simulink model "Boomerang_Simulink_Nav_Kalman"  (R2023a)
settings: Solver=ode4  StartTime=0.0  StopTime=t  FixedStep=dt  MaxStep=maxstep  MinStep=minstep
values from neighbouring files (symbols this model uses):
  c = 5e-2    (= 0.05)    [Boomerang_4Wings.m]    (also in Boomerang_4Wings_Titan.m = 0.0488; Boomerang_4Wings_Venus52.m; Boomerang_4Wings_Venus60.m = 0.065; Boomerang_Cropped_Validation.m = 0.0381)
  CDdata = [x_CD, y_CD]    [Boomerang_4Wings.m]    (also in Boomerang_4Wings_Titan.m; Boomerang_4Wings_Venus52.m; Boomerang_4Wings_Venus60.m; Boomerang_Cropped_Validation.m)
  CLdata = [x_CL, y_CL]    [Boomerang_4Wings.m]    (also in Boomerang_4Wings_Titan.m; Boomerang_4Wings_Venus52.m; Boomerang_4Wings_Venus60.m; Boomerang_Cropped_Validation.m)
  CMdata = [x_CM, y_CM]    [Boomerang_4Wings.m]    (also in Boomerang_4Wings_Titan.m; Boomerang_4Wings_Venus52.m; Boomerang_4Wings_Venus60.m; Boomerang_Cropped_Validation.m)
  dt = 2e-4    (= 0.0002)    [Boomerang_4Wings.m]    (also in Boomerang_4Wings_Titan.m; Boomerang_4Wings_Venus52.m; Boomerang_4Wings_Venus60.m; Boomerang_Cropped_Validation.m)
  Eul0 = [0; 0; 0]    [Boomerang_4Wings.m]    (also in Boomerang_4Wings_Titan.m; Boomerang_4Wings_Venus52.m; Boomerang_4Wings_Venus60.m; Boomerang_Cropped_Validation.m)
  f = 1000    [Boomerang_4Wings.m]    (also in Boomerang_Flight_Dynamics.m; Boomerang_Flight_Dynamics_twisted_wing.m = @(x) -sqrt(abs(Rp^2 - (x-a(2)).^2)) + b(2); Plot_Results.m = @(x) -sqrt(abs(Rp^2 - (x-a(2)).^2)) + b(2); Vassberg.mat = )
  g = 9.81    [Boomerang_4Wings.m]    (also in Boomerang_4Wings_Titan.m = 1.35; Boomerang_4Wings_Venus52.m; Boomerang_4Wings_Venus60.m = 8.87; Boomerang_Cropped_Validation.m)
  h = l_blade/n    (= 0.006)    [Boomerang_Flight_Dynamics.m]    (also in Boomerang_Flight_Dynamics_twisted_wing.m; Vassberg.mat)
  invJ = inv(J)    [Boomerang_4Wings.m]    (also in Boomerang_4Wings_Titan.m; Boomerang_4Wings_Venus52.m; Boomerang_4Wings_Venus60.m; Boomerang_Cropped_Validation.m)
  invTI0 = transpose(TI0)    [AttitudePlot.m]    (also in AttitudePlot_V0.m = T; Boomerang_4Wings.m; Boomerang_4Wings_Titan.m; Boomerang_4Wings_Venus52.m)
  invTj = zeros(3,3,nw)    [Boomerang_4Wings.m]    (also in Boomerang_4Wings_Titan.m; Boomerang_4Wings_Venus52.m; Boomerang_4Wings_Venus60.m; Boomerang_Cropped_Validation.m)
  J = J + (Ji(:,:,i))    [Boomerang_4Wings.m]    (also in Boomerang_4Wings_Titan.m = diag(diag(J)); Boomerang_4Wings_Venus52.m; Boomerang_4Wings_Venus60.m; Boomerang_Cropped_Validation.m = [Ixx Ixy Ixz)
  l_integrate = linspace(0,l_blade,n)    [Boomerang_4Wings.m]    (also in Boomerang_4Wings_Titan.m; Boomerang_4Wings_Venus52.m; Boomerang_4Wings_Venus60.m; Boomerang_Cropped_Validation.m = linspace(l_blade_0,l_blade,n))
  m = m_b    (= 0.2)    [Boomerang_4Wings.m]    (also in Boomerang_4Wings_Titan.m = m_b*eye(3) + m_add; Boomerang_4Wings_Venus52.m = m_b*eye(3) + m_add; Boomerang_4Wings_Venus60.m = m_b*eye(3) + m_add; Boomerang_Cropped_Validation.m = m_b*eye(3) + m_add)
  nw = 4    [Boomerang_4Wings.m]    (also in Boomerang_4Wings_Titan.m; Boomerang_4Wings_Venus52.m; Boomerang_4Wings_Venus60.m; Boomerang_Cropped_Validation.m = 3)
  omega0 = [0; 0; 10*pi*2]    [Boomerang_4Wings.m]    (also in Boomerang_4Wings_Titan.m = [0; 0; r*pi*2]; Boomerang_4Wings_Venus52.m; Boomerang_4Wings_Venus60.m; Boomerang_Cropped_Validation.m = [0; 0; r])
  PHI0 = deg2rad(PHI0)    [AttitudePlot.m]    (also in AttitudePlot_V0.m; Boomerang_4Wings.m; Boomerang_4Wings_Titan.m; Boomerang_4Wings_Venus52.m)
  PSI0 = deg2rad(PSI0)    [AttitudePlot.m]    (also in AttitudePlot_V0.m; Boomerang_4Wings.m; Boomerang_4Wings_Titan.m; Boomerang_4Wings_Venus52.m)
  R_pos0 = [0; 0; 1.5]    [Boomerang_4Wings.m]    (also in Boomerang_4Wings_Titan.m; Boomerang_4Wings_Venus52.m; Boomerang_4Wings_Venus60.m; Boomerang_Cropped_Validation.m = [0; 0; 1.8])
  rho = 1.22    [Boomerang_4Wings.m]    (also in Boomerang_4Wings_Titan.m = 5.368; Boomerang_4Wings_Venus52.m = 1.3288004; Boomerang_4Wings_Venus60.m = 0.49007955; Boomerang_Cropped_Validation.m)
  S = pi*R^2    (= 0.196349540849)    [Boomerang_4Wings.m]    (also in Boomerang_4Wings_Titan.m = 0.228; Boomerang_4Wings_Venus52.m; Boomerang_4Wings_Venus60.m = 0.282743338823; Boomerang_Cropped_Validation.m = 0.0651440652648)
  THETA0 = deg2rad(THETA0)    [AttitudePlot.m]    (also in AttitudePlot_V0.m; Boomerang_4Wings.m; Boomerang_4Wings_Titan.m; Boomerang_4Wings_Venus52.m)
  thetaj = 0    [Boomerang_4Wings.m]    (also in Boomerang_4Wings_Titan.m; Boomerang_4Wings_Venus52.m; Boomerang_4Wings_Venus60.m; Boomerang_Cropped_Validation.m = deg2rad(thetaj))
  TI0 = RI01*RI02*RI03    [AttitudePlot.m]    (also in Boomerang_4Wings.m; Boomerang_4Wings_Titan.m; Boomerang_4Wings_Venus52.m; Boomerang_4Wings_Venus60.m)
  Tj = zeros(3,3, nw)    [Boomerang_4Wings.m]    (also in Boomerang_4Wings_Titan.m; Boomerang_4Wings_Venus52.m; Boomerang_4Wings_Venus60.m; Boomerang_Cropped_Validation.m)
  u0 = TI0*U0    [Boomerang_4Wings.m]    (also in Boomerang_4Wings_Titan.m; Boomerang_4Wings_Venus52.m; Boomerang_4Wings_Venus60.m; Boomerang_Cropped_Validation.m)
  v_wind = [0; 0; 0]    [Boomerang_4Wings.m]    (also in Boomerang_4Wings_Titan.m; Boomerang_4Wings_Venus52.m; Boomerang_4Wings_Venus60.m; Boomerang_Cropped_Validation.m)
  x_ac = zeros(3,nw)    [Boomerang_4Wings.m]    (also in Boomerang_4Wings_Titan.m = 0; Boomerang_4Wings_Venus52.m; Boomerang_4Wings_Venus60.m; Boomerang_Cropped_Validation.m)
undefined symbols (not defined in the file or in its folder): delta_theta, t_action
libraries: simulink_extras x3, aerolibnav x2, sharedTrackingLibrary x2
settings Model: Creator=dsantis  LastModifiedBy=dsantis

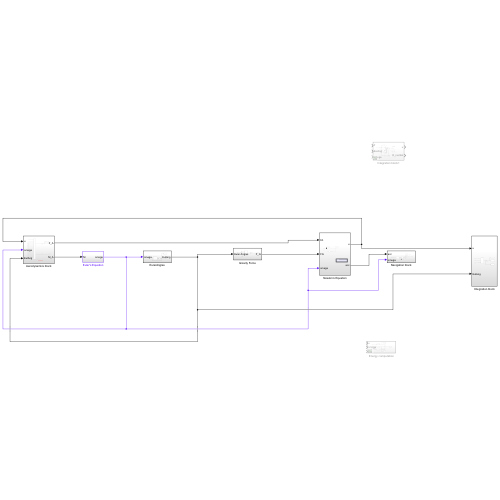
[thumbnail: Simulink's stored preview of the top-level diagram]
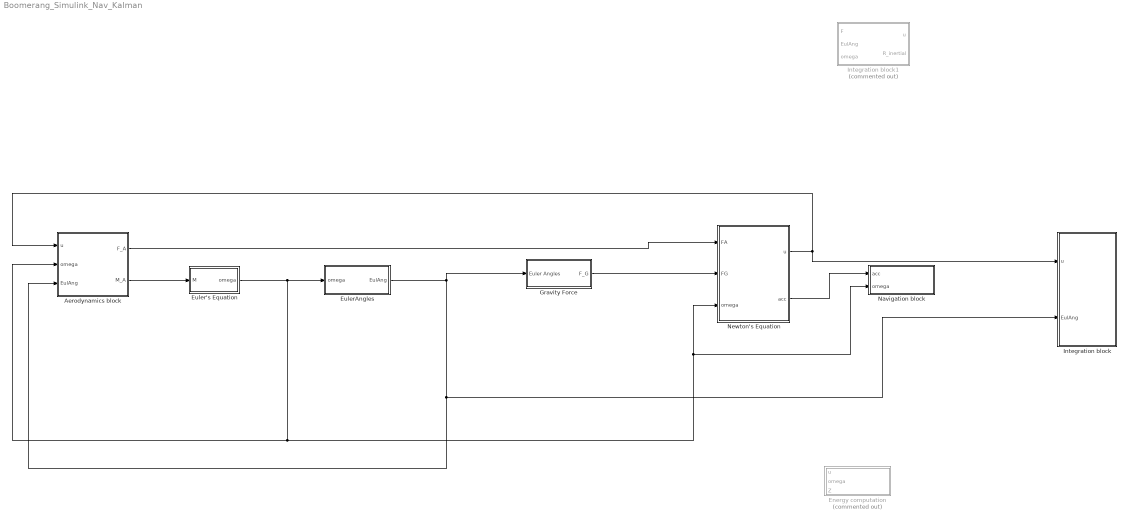
== system Boomerang_Simulink_Nav_Kalman ==
  Aerodynamics block : Subsystem
  Energy computation : Subsystem  Commented=on
  Euler's Equation : Subsystem
  EulerAngles : Subsystem
  Gravity Force : Subsystem
  Integration block : Subsystem
  Integration block1 : Subsystem  Commented=on
  Navigation block : Subsystem
  Newton's Equation : Subsystem
  wires:
  Euler's Equation/1(omega) -> EulerAngles/1(omega), Aerodynamics block/2(omega), Newton's Equation/3(omega), Navigation block/2(omega)
  Newton's Equation/1(u) -> Aerodynamics block/1(u), Integration block/1(u)
  Gravity Force/1(F_G) -> Newton's Equation/2(FG)
  Aerodynamics block/2(M_A) -> Euler's Equation/1(M)
  EulerAngles/1(EulAng) -> Gravity Force/1(Euler Angles), Aerodynamics block/3(EulAng), Integration block/2(EulAng)
  Aerodynamics block/1(F_A) -> Newton's Equation/1(FA)
  Newton's Equation/2(acc) -> Navigation block/1(acc)

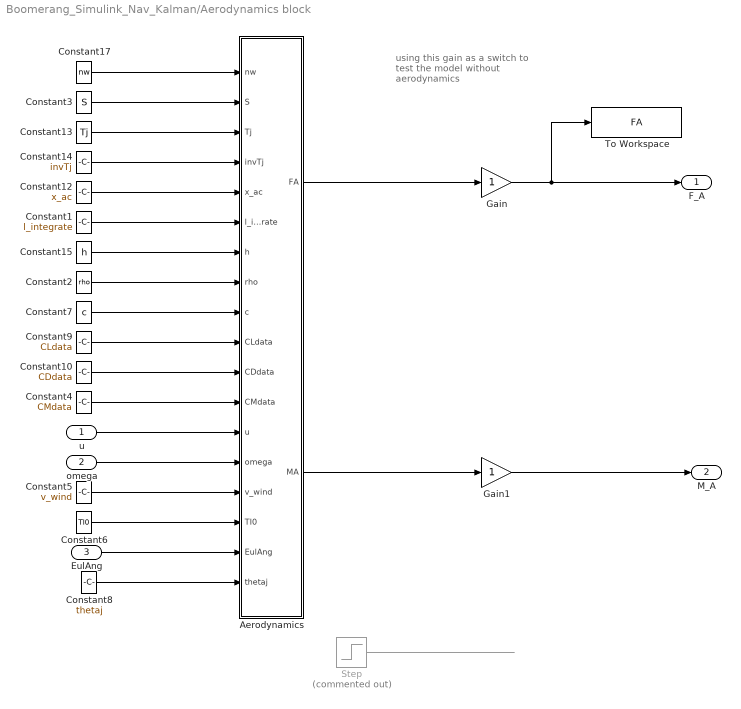
== system Boomerang_Simulink_Nav_Kalman/Aerodynamics block ==
  note: using this gain as a switch
      | to test the model without aerodynamics
  u : Inport
  omega : Inport  Port=2
  EulAng : Inport  Port=3
  Aerodynamics : MATLAB Function  TreatAsAtomicUnit=on
  Constant1 : Constant  Value=l_integrate
  Constant10 : Constant  Value=CDdata
  Constant12 : Constant  Value=x_ac
  Constant13 : Constant  Value=Tj
  Constant14 : Constant  Value=invTj
  Constant15 : Constant  Value=h
  Constant17 : Constant  Value=nw
  Constant2 : Constant  Value=rho
  Constant3 : Constant  Value=S
  Constant4 : Constant  Value=CMdata
  Constant5 : Constant  Value=v_wind
  Constant6 : Constant  Value=TI0
  Constant7 : Constant  Value=c
  Constant8 : Constant  Value=thetaj
  Constant9 : Constant  Value=CLdata
  Gain : Gain
  Gain1 : Gain
  Step : Step  Commented=on  Time=t_action  After=delta_theta  SampleTime=0  VectorParams1D=off
  To Workspace : ToWorkspace  VariableName=FA  SaveFormat=Timeseries  SampleTime=-1
  F_A : Outport
  M_A : Outport  Port=2
  wires:
  u/1 -> Aerodynamics/13(u)
  Constant2/1 -> Aerodynamics/8(rho)
  Constant9/1 -> Aerodynamics/10(CLdata)
  Constant10/1 -> Aerodynamics/11(CDdata)
  Constant1/1 -> Aerodynamics/6(l_integrate)
  Constant7/1 -> Aerodynamics/9(c)
  omega/1 -> Aerodynamics/14(omega)
  Constant12/1 -> Aerodynamics/5(x_ac)
  Constant14/1 -> Aerodynamics/4(invTj)
  Constant13/1 -> Aerodynamics/3(Tj)
  Constant15/1 -> Aerodynamics/7(h)
  Aerodynamics/1(FA) -> Gain/1
  Constant17/1 -> Aerodynamics/1(nw)
  Constant3/1 -> Aerodynamics/2(S)
  Gain/1 -> To Workspace/1, F_A/1
  Constant4/1 -> Aerodynamics/12(CMdata)
  Gain1/1 -> M_A/1
  Step/1 -> ?
  Aerodynamics/2(MA) -> Gain1/1
  Constant5/1 -> Aerodynamics/15(v_wind)
  Constant6/1 -> Aerodynamics/16(TI0)
  EulAng/1 -> Aerodynamics/17(EulAng)
  Constant8/1 -> Aerodynamics/18(thetaj)

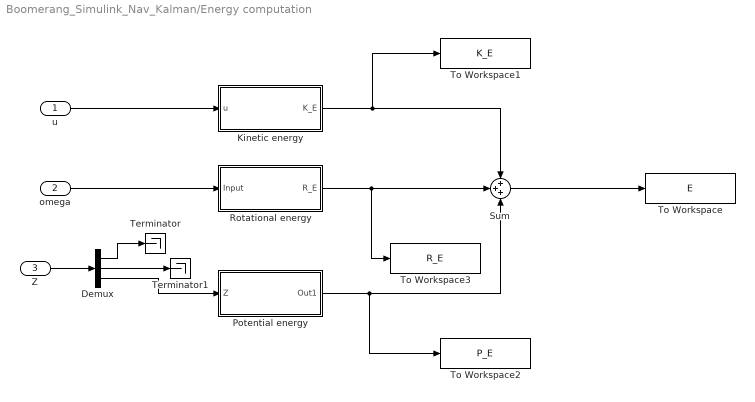
== system Boomerang_Simulink_Nav_Kalman/Energy computation ==
  u : Inport
  omega : Inport  Port=2
  Z : Inport  Port=3
  Demux : Demux  Outputs=3
  Kinetic energy : Subsystem
  Potential energy : Subsystem
  Rotational energy : Subsystem
  Sum : Sum  Inputs=+++
  Terminator : Terminator
  Terminator1 : Terminator
  To Workspace : ToWorkspace  VariableName=E  SaveFormat=Timeseries  SampleTime=-1
  To Workspace1 : ToWorkspace  VariableName=K_E  SaveFormat=Timeseries  SampleTime=-1
  To Workspace2 : ToWorkspace  VariableName=P_E  SaveFormat=Timeseries  SampleTime=-1
  To Workspace3 : ToWorkspace  VariableName=R_E  SaveFormat=Timeseries  SampleTime=-1
  wires:
  u/1 -> Kinetic energy/1(u)
  omega/1 -> Rotational energy/1(Input)
  Z/1 -> Demux/1
  Demux/3 -> Potential energy/1(Z)
  Demux/1 -> Terminator/1
  Demux/2 -> Terminator1/1
  Kinetic energy/1(K_E) -> To Workspace1/1, Sum/1
  Rotational energy/1(R_E) -> To Workspace3/1, Sum/2
  Potential energy/1(Out1) -> To Workspace2/1, Sum/3
  Sum/1 -> To Workspace/1

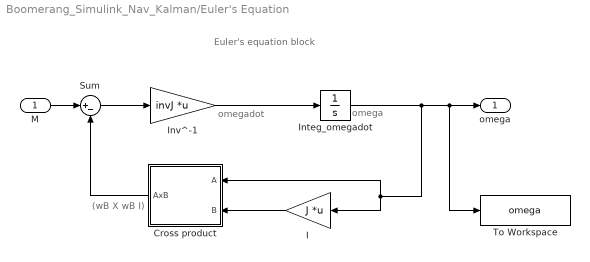
== system Boomerang_Simulink_Nav_Kalman/Euler's Equation ==
  note: Euler's equation block
  note: (wB X wB I)
  note: omega
  note: omegadot
  M : Inport
  Cross product : Subsystem
  I : Gain  Gain=J  Multiplication=Matrix(K*u)
  Integ_omegadot : Integrator  InitialCondition=omega0
  Inv^-1 : Gain  Gain=invJ  Multiplication=Matrix(K*u) (u vector)
  Sum : Sum  Inputs=|+-
  To Workspace : ToWorkspace  VariableName=omega  SampleTime=-1
  omega : Outport  VectorParamsAs1DForOutWhenUnconnected=off
  wires:
  Integ_omegadot/1 -> To Workspace/1, omega/1, I/1, Cross product/1(A)
  I/1 -> Cross product/2(B)
  M/1 -> Sum/1
  Sum/1 -> Inv^-1/1
  Inv^-1/1 -> Integ_omegadot/1
  Cross product/1(AxB) -> Sum/2

== system Boomerang_Simulink_Nav_Kalman/EulerAngles ==
  omega : Inport
  Integrator : Integrator  InitialCondition=Eul0
  MATLAB Function : MATLAB Function  TreatAsAtomicUnit=on
  To Workspace : ToWorkspace  VariableName=EulAng  SampleTime=-1
  EulAng : Outport
  wires:
  omega/1 -> MATLAB Function/1(omega)
  MATLAB Function/1(EulRate) -> Integrator/1
  Integrator/1 -> MATLAB Function/2(EulAng), EulAng/1, To Workspace/1

== system Boomerang_Simulink_Nav_Kalman/Gravity Force ==
  Euler Angles : Inport
  Constant : Constant  Value=TI0
  Demux : Demux  Outputs=3
  Gain : Gain  Gain=-m*g
  MATLAB Function : MATLAB Function  TreatAsAtomicUnit=on
  F_G : Outport
  wires:
  Gain/1 -> F_G/1
  Demux/3 -> MATLAB Function/3(psi)
  Demux/2 -> MATLAB Function/2(theta)
  Demux/1 -> MATLAB Function/1(phi)
  MATLAB Function/1(CG) -> Gain/1
  Euler Angles/1 -> Demux/1
  Constant/1 -> MATLAB Function/4(TI0)

== system Boomerang_Simulink_Nav_Kalman/Integration block ==
  u : Inport
  EulAng : Inport  Port=2
  Body2Inertial : MATLAB Function  TreatAsAtomicUnit=on
  Constant : Constant  Value=invTI0
  Integrator1 : Integrator  InitialCondition=R_pos0
  Stop if Z < 0 : Subsystem
  To Workspace : ToWorkspace  VariableName=U  SampleTime=-1
  To Workspace1 : ToWorkspace  VariableName=R_inertial  SampleTime=-1
  wires:
  Integrator1/1 -> Stop if Z < 0/1(R_inertial), To Workspace1/1
  Body2Inertial/1(U) -> To Workspace/1, Integrator1/1
  u/1 -> Body2Inertial/1(u)
  Constant/1 -> Body2Inertial/3(invTI0)
  EulAng/1 -> Body2Inertial/2(EulAng)

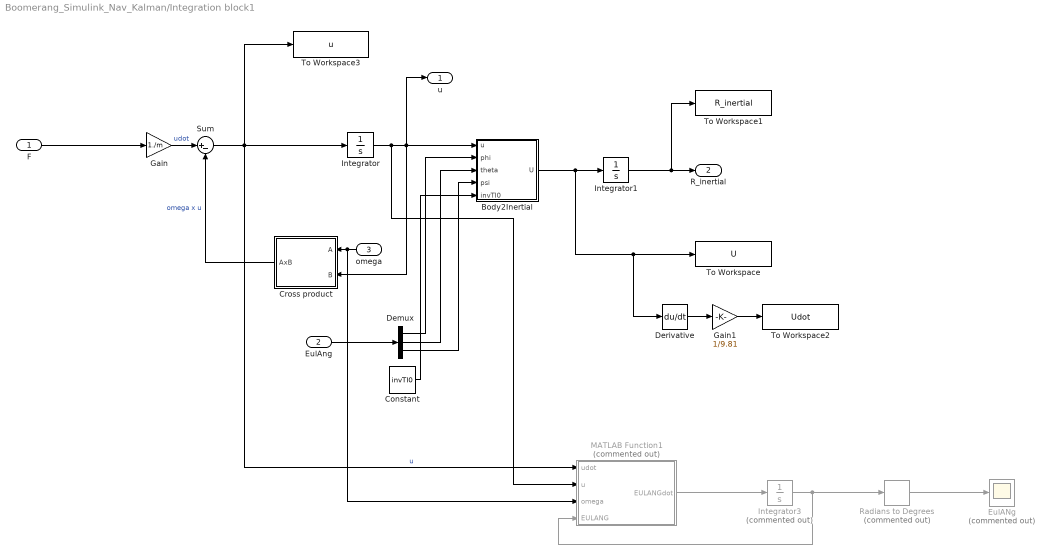
== system Boomerang_Simulink_Nav_Kalman/Integration block1 ==
  F : Inport
  EulAng : Inport  Port=2
  omega : Inport  Port=3
  Body2Inertial : MATLAB Function  TreatAsAtomicUnit=on
  Constant : Constant  Value=invTI0
  Cross product : Subsystem
  Demux : Demux  Outputs=3
  Derivative : Derivative
  EulANg : Scope  Commented=on
  Gain : Gain  Gain=1./m
  Gain1 : Gain  Gain=1/9.81
  Integrator : Integrator  InitialCondition=u0
  Integrator1 : Integrator  InitialCondition=R_pos0
  Integrator3 : Integrator  Commented=on  InitialCondition=[PHI0; THETA0; PSI0]
  MATLAB Function1 : MATLAB Function  Commented=on  TreatAsAtomicUnit=on
  Radians to Degrees : simulink_extras/Transformations/Radians to Degrees  Commented=on
  Sum : Sum  Inputs=|+-
  To Workspace : ToWorkspace  VariableName=U  SampleTime=-1
  To Workspace1 : ToWorkspace  VariableName=R_inertial  SampleTime=-1
  To Workspace2 : ToWorkspace  VariableName=Udot  SaveFormat=Timeseries  SampleTime=-1
  To Workspace3 : ToWorkspace  VariableName=u  SampleTime=-1
  u : Outport
  R_inertial : Outport  Port=2
  wires:
  Cross product/1(AxB) -> Sum/2  "omega x u"
  Integrator/1 -> Cross product/2(B), Body2Inertial/1(u), u/1, MATLAB Function1/2(u)
  Integrator1/1 -> To Workspace1/1, R_inertial/1
  Gain/1 -> Sum/1  "udot"
  EulAng/1 -> Demux/1
  Demux/1 -> Body2Inertial/2(phi)
  Demux/2 -> Body2Inertial/3(theta)
  Demux/3 -> Body2Inertial/4(psi)
  Constant/1 -> Body2Inertial/5(invTI0)
  F/1 -> Gain/1
  Body2Inertial/1(U) -> Derivative/1, To Workspace/1, Integrator1/1
  Sum/1 -> To Workspace3/1, MATLAB Function1/1(udot), Integrator/1  "u"
  MATLAB Function1/1(EULANGdot) -> Integrator3/1
  Integrator3/1 -> Radians to Degrees/1, MATLAB Function1/4(EULANG)
  Radians to Degrees/1 -> EulANg/1
  Derivative/1 -> Gain1/1
  Gain1/1 -> To Workspace2/1
  omega/1 -> MATLAB Function1/3(omega), Cross product/1(A)

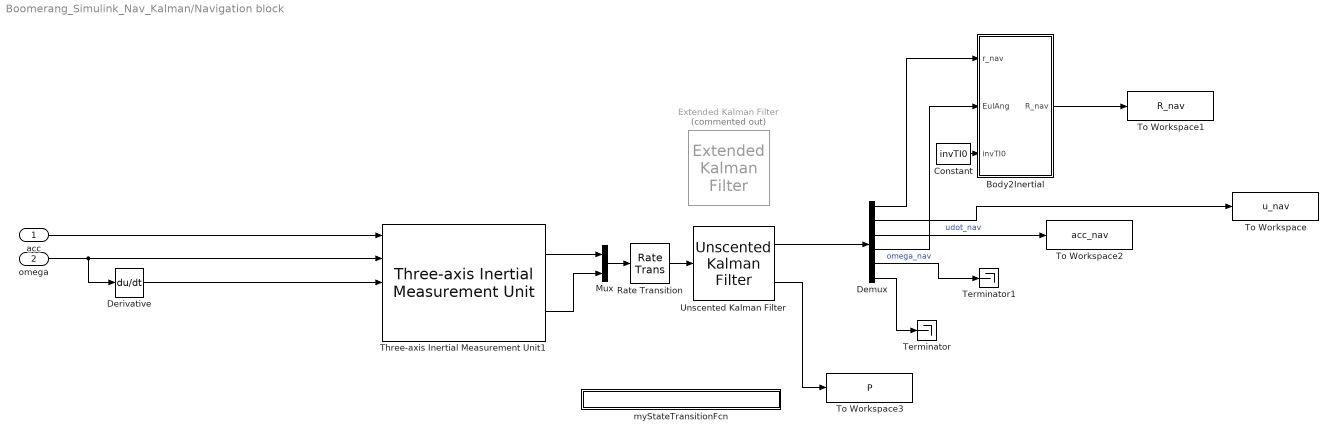
== system Boomerang_Simulink_Nav_Kalman/Navigation block ==
  acc : Inport
  omega : Inport  Port=2
  Body2Inertial : MATLAB Function  TreatAsAtomicUnit=on
  Constant : Constant  Value=invTI0
  Demux : Demux  Outputs=6
  Derivative : Derivative
  Extended Kalman Filter : sharedTrackingLibrary/Extended Kalman Filter  Commented=on  StateTransitionFcn=myStateTransitionFcn  HasStateTransitionJacobianFcn=off  HasAdditiveProcessNoise=Additive  ProcessNoise=diag(ones(18,1))  HasTimeVaryingProcessNoise=off  HasStateTransitionFcnExtraArgument=0  InitialState=[TI0*R_pos0; u0; 0; 0; 0; Eul0; omega0; 0; 0; 0]  InitialStateCovariance=diag(ones(18,1))  MeasurementFcn1=myMeasurementFcn  HasMeasurementJacobianFcn1=off  HasMeasurementEnablePort1=off  HasAdditiveMeasurementNoise1=Additive  MeasurementNoise1=[1 1 1 1 1 1]  HasTimeVaryingMeasurementNoise1=off  HasMeasurementFcnExtraArgument1=0  HasMeasurementWrapping1=off  MeasurementFcn2=myMeasurementFcn  HasMeasurementJacobianFcn2=off  HasMeasurementEnablePort2=off  HasAdditiveMeasurementNoise2=Additive  MeasurementNoise2=1  HasTimeVaryingMeasurementNoise2=off  HasMeasurementFcnExtraArgument2=0  HasMeasurementWrapping2=off  MeasurementFcn3=myMeasurementFcn  HasMeasurementJacobianFcn3=off  HasMeasurementEnablePort3=off  HasAdditiveMeasurementNoise3=Additive  MeasurementNoise3=1  HasTimeVaryingMeasurementNoise3=off  HasMeasurementFcnExtraArgument3=0  HasMeasurementWrapping3=off  MeasurementFcn4=myMeasurementFcn  HasMeasurementJacobianFcn4=off  HasMeasurementEnablePort4=off  HasAdditiveMeasurementNoise4=Additive  MeasurementNoise4=1  HasTimeVaryingMeasurementNoise4=off  HasMeasurementFcnExtraArgument4=0  HasMeasurementWrapping4=off  MeasurementFcn5=myMeasurementFcn  HasMeasurementJacobianFcn5=off  HasMeasurementEnablePort5=off  HasAdditiveMeasurementNoise5=Additive  MeasurementNoise5=1  HasTimeVaryingMeasurementNoise5=off  HasMeasurementFcnExtraArgument5=0  HasMeasurementWrapping5=off  EnableMultirate=on  StateTransitionFcnSampleTime=1/f  MeasurementFcn1SampleTime=1/f  MeasurementFcn2SampleTime=1  MeasurementFcn3SampleTime=1  MeasurementFcn4SampleTime=1  MeasurementFcn5SampleTime=1  UseCurrentEstimator=on  OutputStateCovariance=off  DataType=double  SampleTime=1  NumberOfMeasurements=1
  Mux : Mux  Inputs=2
  Rate Transition : RateTransition
  Terminator : Terminator
  Terminator1 : Terminator
  Three-axis Inertial Measurement Unit1 : aerolibnav/Three-axis Inertial Measurement Unit  units=Metric (MKS)  imu=[0 0 0]  i_Ts=0  dtype_a=off  w_a=190  z_a=0.707  a_sf_cc=acc.sf  a_bias=acc.bias  a_sat=acc.lim  dtype_g=off  w_g=190  z_g=0.707  g_sf_cc=gyro.sf  g_bias=gyro.bias  g_sens=gyro.gbias  g_sat=gyro.lim  i_rand=on  i_seeds=[23093 23094 23095 23096 23097 23098]  i_pow=noise
  To Workspace : ToWorkspace  VariableName=u_nav  SampleTime=-1
  To Workspace1 : ToWorkspace  VariableName=R_nav  SampleTime=-1
  To Workspace2 : ToWorkspace  VariableName=acc_nav  SampleTime=-1
  To Workspace3 : ToWorkspace  VariableName=P  SampleTime=-1
  Unscented Kalman Filter : sharedTrackingLibrary/Unscented Kalman Filter  StateTransitionFcn=myStateTransitionFcn  HasAdditiveProcessNoise=Additive  ProcessNoise=diag(ones(18,1))  HasTimeVaryingProcessNoise=off  HasStateTransitionFcnExtraArgument=0  InitialState=[TI0*R_pos0; u0; 0; 0; 0; Eul0; omega0; 0; 0; 0]  InitialStateCovariance=diag(ones(18,1))  Alpha=1e-3  Beta=2  Kappa=0  MeasurementFcn1=myMeasurementFcn  HasMeasurementEnablePort1=off  HasAdditiveMeasurementNoise1=Additive  MeasurementNoise1=[0.0001 0.0001 0.0001 0.0001 0.0001 0.0001]  HasTimeVaryingMeasurementNoise1=off  HasMeasurementFcnExtraArgument1=0  HasMeasurementWrapping1=off  MeasurementFcn2=myMeasurementFcn  HasMeasurementEnablePort2=off  HasAdditiveMeasurementNoise2=Additive  MeasurementNoise2=1  HasTimeVaryingMeasurementNoise2=off  HasMeasurementFcnExtraArgument2=0  HasMeasurementWrapping2=off  MeasurementFcn3=myMeasurementFcn  HasMeasurementEnablePort3=off  HasAdditiveMeasurementNoise3=Additive  MeasurementNoise3=1  HasTimeVaryingMeasurementNoise3=off  HasMeasurementFcnExtraArgument3=0  HasMeasurementWrapping3=off  MeasurementFcn4=myMeasurementFcn  HasMeasurementEnablePort4=off  HasAdditiveMeasurementNoise4=Additive  MeasurementNoise4=1  HasTimeVaryingMeasurementNoise4=off  HasMeasurementFcnExtraArgument4=0  HasMeasurementWrapping4=off  MeasurementFcn5=myMeasurementFcn  HasMeasurementEnablePort5=off  HasAdditiveMeasurementNoise5=Additive  MeasurementNoise5=1  HasTimeVaryingMeasurementNoise5=off  HasMeasurementFcnExtraArgument5=0  HasMeasurementWrapping5=off  EnableMultirate=on  StateTransitionFcnSampleTime=1/f  MeasurementFcn1SampleTime=1/f  MeasurementFcn2SampleTime=1  MeasurementFcn3SampleTime=1  MeasurementFcn4SampleTime=1  MeasurementFcn5SampleTime=1  UseCurrentEstimator=on  OutputStateCovariance=on  DataType=double  SampleTime=1  NumberOfMeasurements=1
      settings: LibrarySourceBlock=cstblocks/State Estimation/Unscented Kalman Filter
  myStateTransitionFcn : Subsystem  TreatAsAtomicUnit=on
  wires:
  Derivative/1 -> Three-axis Inertial Measurement Unit1/3
  acc/1 -> Three-axis Inertial Measurement Unit1/1
  Demux/3 -> To Workspace2/1  "udot_nav"
  omega/1 -> Three-axis Inertial Measurement Unit1/2, Derivative/1
  Demux/6 -> Terminator/1
  Demux/4 -> Body2Inertial/2(EulAng)
  Demux/1 -> Body2Inertial/1(r_nav)
  Demux/2 -> To Workspace/1
  Three-axis Inertial Measurement Unit1/1 -> Mux/1
  Three-axis Inertial Measurement Unit1/2 -> Mux/2
  Mux/1 -> Rate Transition/1
  Constant/1 -> Body2Inertial/3(invTI0)
  Body2Inertial/1(R_nav) -> To Workspace1/1
  Demux/5 -> Terminator1/1  "omega_nav"
  Rate Transition/1 -> Unscented Kalman Filter/1
  Unscented Kalman Filter/2 -> To Workspace3/1
  Unscented Kalman Filter/1 -> Demux/1

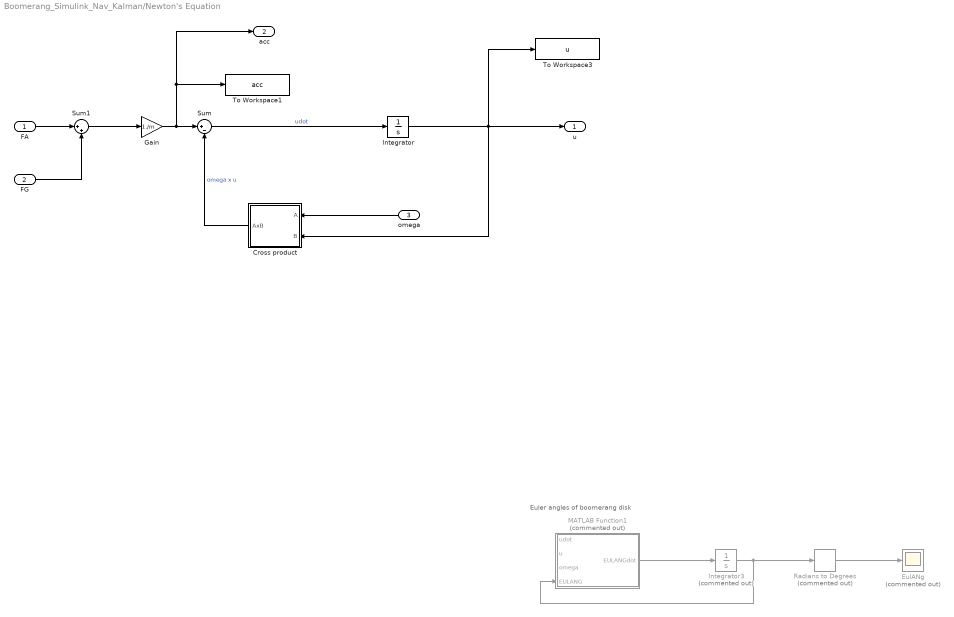
== system Boomerang_Simulink_Nav_Kalman/Newton's Equation ==
  note: Euler angles of boomerang disk
  FA : Inport
  FG : Inport  Port=2
  omega : Inport  Port=3
  Cross product : Subsystem
  EulANg : Scope  Commented=on
  Gain : Gain  Gain=1./m
  Integrator : Integrator  InitialCondition=u0
  Integrator3 : Integrator  Commented=on  InitialCondition=[PHI0; THETA0; PSI0]
  MATLAB Function1 : MATLAB Function  Commented=on  TreatAsAtomicUnit=on
  Radians to Degrees : simulink_extras/Transformations/Radians to Degrees  Commented=on
  Sum : Sum  Inputs=|+-
  Sum1 : Sum  Inputs=|++
  To Workspace1 : ToWorkspace  VariableName=acc  SampleTime=-1
  To Workspace3 : ToWorkspace  VariableName=u  SampleTime=-1
  u : Outport
  acc : Outport  Port=2
  wires:
  Cross product/1(AxB) -> Sum/2  "omega x u"
  Gain/1 -> acc/1, To Workspace1/1, Sum/1
  FA/1 -> Sum1/1
  Sum/1 -> Integrator/1  "udot"
  MATLAB Function1/1(EULANGdot) -> Integrator3/1
  Integrator3/1 -> Radians to Degrees/1, MATLAB Function1/4(EULANG)
  Radians to Degrees/1 -> EulANg/1
  omega/1 -> Cross product/1(A)
  FG/1 -> Sum1/2
  Sum1/1 -> Gain/1
  Integrator/1 -> Cross product/2(B), To Workspace3/1, u/1

== system Boomerang_Simulink_Nav_Kalman/Energy computation/Kinetic energy ==
  u : Inport
  Gain : Gain  Gain=0.5*m
  Norm : MATLAB Function  TreatAsAtomicUnit=on
  K_E : Outport
  wires:
  u/1 -> Norm/1(u)
  Norm/1(y) -> Gain/1
  Gain/1 -> K_E/1

== system Boomerang_Simulink_Nav_Kalman/Energy computation/Potential energy ==
  Z : Inport
  Gain : Gain  Gain=m*g
  Out1 : Outport
  wires:
  Z/1 -> Gain/1
  Gain/1 -> Out1/1

== system Boomerang_Simulink_Nav_Kalman/Energy computation/Rotational energy ==
  Input : Inport
  Dot Product : DotProduct  OutDataTypeStr=Inherit: Inherit via internal rule
  Gain : Gain  Gain=0.5*J  Multiplication=Matrix(u*K)
  R_E : Outport
  wires:
  Input/1 -> Dot Product/2, Gain/1
  Gain/1 -> Dot Product/1
  Dot Product/1 -> R_E/1

== system Boomerang_Simulink_Nav_Kalman/Euler's Equation/Cross product ==
  A : Inport
  B : Inport  Port=2
  MATLAB Fcn : MATLABFcn  MATLABFcn=cross(u(1:3),u(4:6))
  Mux : Mux  Inputs=2
  AxB : Outport  VectorParamsAs1DForOutWhenUnconnected=off
  wires:
  A/1 -> Mux/1
  B/1 -> Mux/2
  Mux/1 -> MATLAB Fcn/1
  MATLAB Fcn/1 -> AxB/1

== system Boomerang_Simulink_Nav_Kalman/Integration block/Stop if Z < 0 ==
  R_inertial : Inport
  Constant : Constant  Value=0
  Demux1 : Demux  Outputs=3
  Relational Operator : RelationalOperator  Operator=<=  OutDataTypeStr=boolean  RndMeth=Simplest  InputSameDT=off
  Stop Simulation : Stop
  Terminator1 : Terminator
  Terminator2 : Terminator
  Three-axis Accelerometer : aerolibnav/Three-axis Accelerometer  units=Metric (MKS)  acc=[0 0 0]  gtype=on  dtype_a=on  w_a=190  z_a=0.707  a_sf_cc=[1 0 0; 0 1 0; 0 0 1]  a_bias=[0 0 0]  a_Ts=0  a_rand=on  a_seeds=[23093 23094 23095]  a_pow=[0.001 0.001 0.001]  a_sat="[-inf  -inf  -inf  inf inf inf]"
  wires:
  R_inertial/1 -> Demux1/1
  Demux1/1 -> Terminator1/1
  Demux1/3 -> Relational Operator/1
  Demux1/2 -> Terminator2/1
  Constant/1 -> Relational Operator/2
  Relational Operator/1 -> Stop Simulation/1

== system Boomerang_Simulink_Nav_Kalman/Integration block1/Cross product ==
  A : Inport
  B : Inport  Port=2
  MATLAB Fcn : MATLABFcn  MATLABFcn=cross(u(1:3),u(4:6))
  Mux : Mux  Inputs=2
  AxB : Outport  VectorParamsAs1DForOutWhenUnconnected=off
  wires:
  A/1 -> Mux/1
  B/1 -> Mux/2
  Mux/1 -> MATLAB Fcn/1
  MATLAB Fcn/1 -> AxB/1

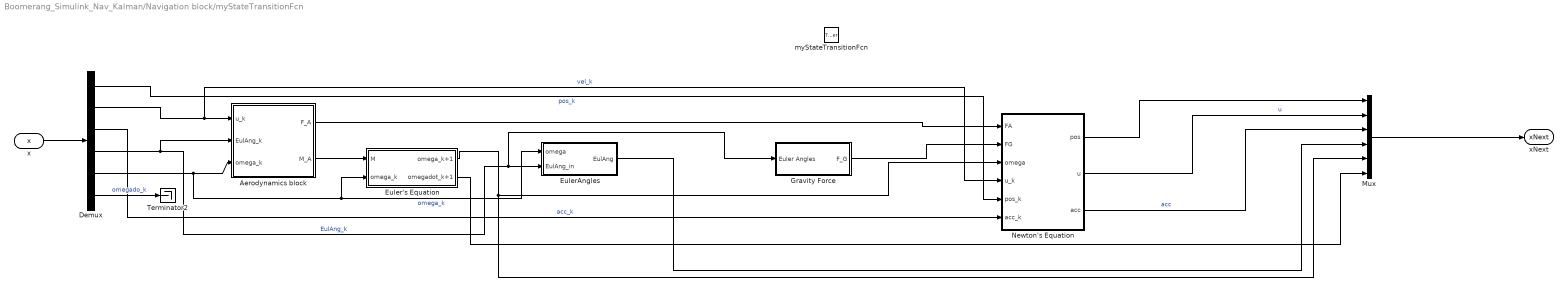
== system Boomerang_Simulink_Nav_Kalman/Navigation block/myStateTransitionFcn ==
  myStateTransitionFcn : TriggerPort  TriggerType=function-call  IsSimulinkFunction=on  FunctionName=myStateTransitionFcn  FunctionVisibility=scoped  VariantControl=(inherit)
  Aerodynamics block : Subsystem
  Demux : Demux  Outputs=6
  Euler's Equation : Subsystem
  EulerAngles : Subsystem
  Gravity Force : Subsystem
  Mux : Mux  Inputs=6
  Newton's Equation : Subsystem
  Terminator2 : Terminator
  x : ArgIn  DisableCoverage=on  PortDimensions=18  ArgumentName=x
  xNext : ArgOut  DisableCoverage=on  PortDimensions=18  ArgumentName=xNext
  wires:
  x/1 -> Demux/1
  Gravity Force/1(F_G) -> Newton's Equation/2(FG)
  EulerAngles/1(EulAng) -> Mux/4
  Aerodynamics block/1(F_A) -> Newton's Equation/1(FA)
  Aerodynamics block/2(M_A) -> Euler's Equation/1(M)
  Euler's Equation/1(omega_k+1) -> Newton's Equation/3(omega), Mux/5
  Mux/1 -> xNext/1
  Demux/1 -> Newton's Equation/5(pos_k)  "pos_k"
  Demux/2 -> Newton's Equation/4(u_k), Aerodynamics block/1(u_k)  "vel_k"
  Demux/4 -> Gravity Force/1(Euler Angles), EulerAngles/2(EulAng_in), Aerodynamics block/2(EulAng_k)  "EulAng_k"
  Demux/5 -> EulerAngles/1(omega), Euler's Equation/2(omega_k), Aerodynamics block/3(omega_k)  "omega_k"
  Demux/3 -> Newton's Equation/6(acc_k)  "acc_k"
  Demux/6 -> Terminator2/1  "omegado_k"
  Euler's Equation/2(omegadot_k+1) -> Mux/6
  Newton's Equation/2(u) -> Mux/2  "u"
  Newton's Equation/3(acc) -> Mux/3  "acc"
  Newton's Equation/1(pos) -> Mux/1

== system Boomerang_Simulink_Nav_Kalman/Newton's Equation/Cross product ==
  A : Inport
  B : Inport  Port=2
  MATLAB Fcn : MATLABFcn  MATLABFcn=cross(u(1:3),u(4:6))
  Mux : Mux  Inputs=2
  AxB : Outport  VectorParamsAs1DForOutWhenUnconnected=off
  wires:
  A/1 -> Mux/1
  B/1 -> Mux/2
  Mux/1 -> MATLAB Fcn/1
  MATLAB Fcn/1 -> AxB/1

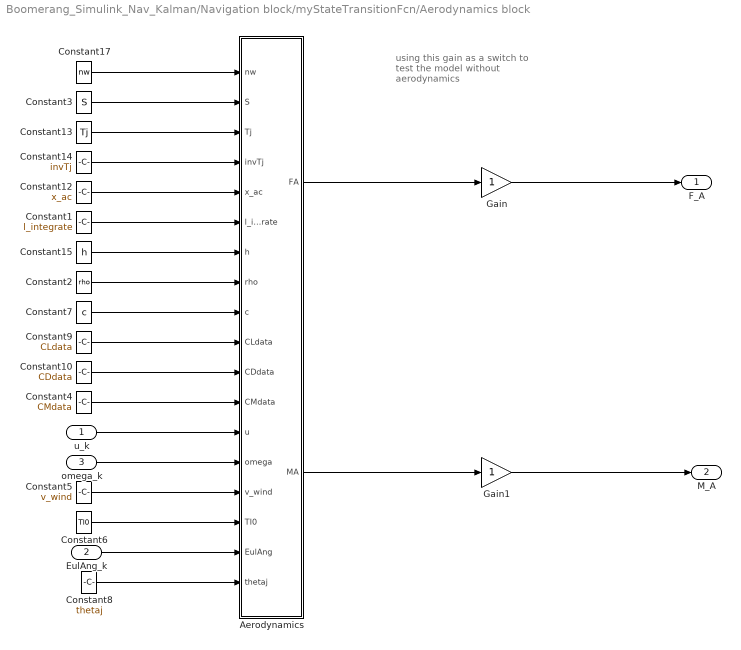
== system Boomerang_Simulink_Nav_Kalman/Navigation block/myStateTransitionFcn/Aerodynamics block ==
  note: using this gain as a switch
      | to test the model without aerodynamics
  u_k : Inport
  EulAng_k : Inport  Port=2
  omega_k : Inport  Port=3
  Aerodynamics : MATLAB Function  TreatAsAtomicUnit=on
  Constant1 : Constant  Value=l_integrate
  Constant10 : Constant  Value=CDdata
  Constant12 : Constant  Value=x_ac
  Constant13 : Constant  Value=Tj
  Constant14 : Constant  Value=invTj
  Constant15 : Constant  Value=h
  Constant17 : Constant  Value=nw
  Constant2 : Constant  Value=rho
  Constant3 : Constant  Value=S
  Constant4 : Constant  Value=CMdata
  Constant5 : Constant  Value=v_wind
  Constant6 : Constant  Value=TI0
  Constant7 : Constant  Value=c
  Constant8 : Constant  Value=thetaj
  Constant9 : Constant  Value=CLdata
  Gain : Gain
  Gain1 : Gain
  F_A : Outport
  M_A : Outport  Port=2
  wires:
  u_k/1 -> Aerodynamics/13(u)
  Constant2/1 -> Aerodynamics/8(rho)
  Constant9/1 -> Aerodynamics/10(CLdata)
  Constant10/1 -> Aerodynamics/11(CDdata)
  Constant1/1 -> Aerodynamics/6(l_integrate)
  Constant7/1 -> Aerodynamics/9(c)
  omega_k/1 -> Aerodynamics/14(omega)
  Constant12/1 -> Aerodynamics/5(x_ac)
  Constant14/1 -> Aerodynamics/4(invTj)
  Constant13/1 -> Aerodynamics/3(Tj)
  Constant15/1 -> Aerodynamics/7(h)
  Aerodynamics/1(FA) -> Gain/1
  Constant17/1 -> Aerodynamics/1(nw)
  Constant3/1 -> Aerodynamics/2(S)
  Gain/1 -> F_A/1
  Constant4/1 -> Aerodynamics/12(CMdata)
  Gain1/1 -> M_A/1
  Aerodynamics/2(MA) -> Gain1/1
  Constant5/1 -> Aerodynamics/15(v_wind)
  Constant6/1 -> Aerodynamics/16(TI0)
  EulAng_k/1 -> Aerodynamics/17(EulAng)
  Constant8/1 -> Aerodynamics/18(thetaj)

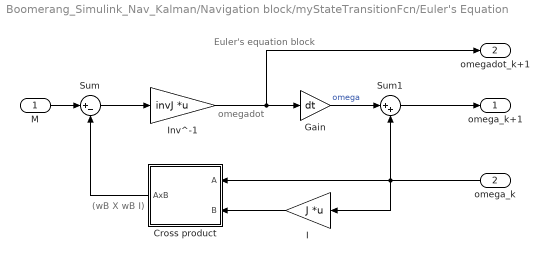
== system Boomerang_Simulink_Nav_Kalman/Navigation block/myStateTransitionFcn/Euler's Equation ==
  note: Euler's equation block
  note: (wB X wB I)
  note: omegadot
  M : Inport
  omega_k : Inport  Port=2
  Cross product : Subsystem
  Gain : Gain  Gain=dt
  I : Gain  Gain=J  Multiplication=Matrix(K*u)
  Inv^-1 : Gain  Gain=invJ  Multiplication=Matrix(K*u) (u vector)
  Sum : Sum  Inputs=|+-
  Sum1 : Sum  Inputs=|++
  omega_k+1 : Outport  VectorParamsAs1DForOutWhenUnconnected=off
  omegadot_k+1 : Outport  Port=2
  wires:
  Gain/1 -> Sum1/1  "omega"
  I/1 -> Cross product/2(B)
  M/1 -> Sum/1
  Sum/1 -> Inv^-1/1
  Inv^-1/1 -> Gain/1, omegadot_k+1/1
  Cross product/1(AxB) -> Sum/2
  omega_k/1 -> Cross product/1(A), I/1, Sum1/2
  Sum1/1 -> omega_k+1/1

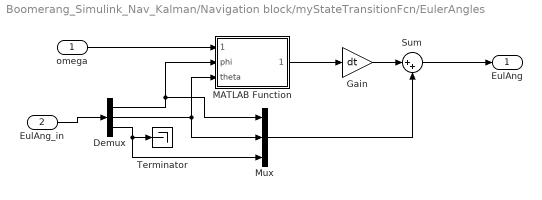
== system Boomerang_Simulink_Nav_Kalman/Navigation block/myStateTransitionFcn/EulerAngles ==
  omega : Inport
  EulAng_in : Inport  Port=2
  Demux : Demux  Outputs=3
  Gain : Gain  Gain=dt
  MATLAB Function : MATLAB Function  TreatAsAtomicUnit=on
  Mux : Mux  Inputs=3
  Sum : Sum  Inputs=|++
  Terminator : Terminator
  EulAng : Outport
  wires:
  omega/1 -> MATLAB Function/1(omega)
  MATLAB Function/1(EulRate) -> Gain/1
  Sum/1 -> EulAng/1
  EulAng_in/1 -> Demux/1
  Demux/1 -> MATLAB Function/2(phi), Mux/1
  Demux/2 -> MATLAB Function/3(theta), Mux/2
  Demux/3 -> Mux/3, Terminator/1
  Gain/1 -> Sum/1
  Mux/1 -> Sum/2

== system Boomerang_Simulink_Nav_Kalman/Navigation block/myStateTransitionFcn/Gravity Force ==
  Euler Angles : Inport
  Constant : Constant  Value=TI0
  Demux : Demux  Outputs=3
  Gain : Gain  Gain=-m*g
  MATLAB Function : MATLAB Function  TreatAsAtomicUnit=on
  F_G : Outport
  wires:
  Gain/1 -> F_G/1
  Demux/3 -> MATLAB Function/3(psi)
  Demux/2 -> MATLAB Function/2(theta)
  Demux/1 -> MATLAB Function/1(phi)
  MATLAB Function/1(CG) -> Gain/1
  Euler Angles/1 -> Demux/1
  Constant/1 -> MATLAB Function/4(TI0)

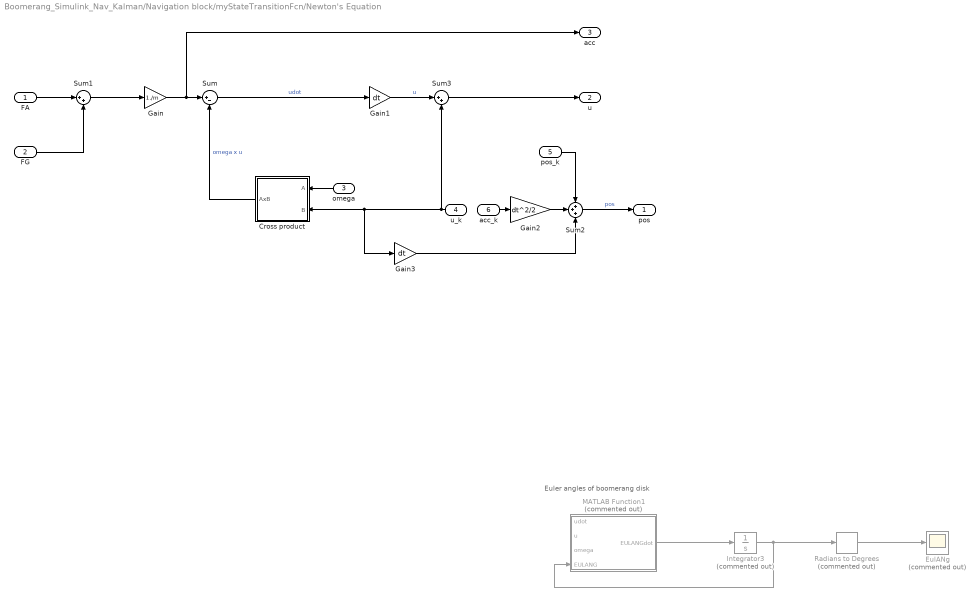
== system Boomerang_Simulink_Nav_Kalman/Navigation block/myStateTransitionFcn/Newton's Equation ==
  note: Euler angles of boomerang disk
  FA : Inport
  FG : Inport  Port=2
  omega : Inport  Port=3
  u_k : Inport  Port=4
  pos_k : Inport  Port=5
  acc_k : Inport  Port=6
  Cross product : Subsystem
  EulANg : Scope  Commented=on
  Gain : Gain  Gain=1./m
  Gain1 : Gain  Gain=dt
  Gain2 : Gain  Gain=dt^2/2
  Gain3 : Gain  Gain=dt
  Integrator3 : Integrator  Commented=on  InitialCondition=[PHI0; THETA0; PSI0]
  MATLAB Function1 : MATLAB Function  Commented=on  TreatAsAtomicUnit=on
  Radians to Degrees : simulink_extras/Transformations/Radians to Degrees  Commented=on
  Sum : Sum  Inputs=|+-
  Sum1 : Sum  Inputs=|++
  Sum2 : Sum  Inputs=+++
  Sum3 : Sum  Inputs=|++
  pos : Outport
  u : Outport  Port=2
  acc : Outport  Port=3
  wires:
  Cross product/1(AxB) -> Sum/2  "omega x u"
  Gain/1 -> acc/1, Sum/1
  FA/1 -> Sum1/1
  Sum/1 -> Gain1/1  "udot"
  MATLAB Function1/1(EULANGdot) -> Integrator3/1
  Integrator3/1 -> Radians to Degrees/1, MATLAB Function1/4(EULANG)
  Radians to Degrees/1 -> EulANg/1
  omega/1 -> Cross product/1(A)
  FG/1 -> Sum1/2
  Sum1/1 -> Gain/1
  Sum2/1 -> pos/1  "pos"
  u_k/1 -> Sum3/2, Gain3/1, Cross product/2(B)
  pos_k/1 -> Sum2/1
  Gain1/1 -> Sum3/1  "u"
  Sum3/1 -> u/1
  Gain2/1 -> Sum2/2
  Gain3/1 -> Sum2/3
  acc_k/1 -> Gain2/1

== system Boomerang_Simulink_Nav_Kalman/Navigation block/myStateTransitionFcn/Euler's Equation/Cross product ==
  A : Inport
  B : Inport  Port=2
  MATLAB Fcn : MATLABFcn  MATLABFcn=cross(u(1:3),u(4:6))
  Mux : Mux  Inputs=2
  AxB : Outport  VectorParamsAs1DForOutWhenUnconnected=off
  wires:
  A/1 -> Mux/1
  B/1 -> Mux/2
  Mux/1 -> MATLAB Fcn/1
  MATLAB Fcn/1 -> AxB/1

== system Boomerang_Simulink_Nav_Kalman/Navigation block/myStateTransitionFcn/Newton's Equation/Cross product ==
  A : Inport
  B : Inport  Port=2
  MATLAB Fcn : MATLABFcn  MATLABFcn=cross(u(1:3),u(4:6))
  Mux : Mux  Inputs=2
  AxB : Outport  VectorParamsAs1DForOutWhenUnconnected=off
  wires:
  A/1 -> Mux/1
  B/1 -> Mux/2
  Mux/1 -> MATLAB Fcn/1
  MATLAB Fcn/1 -> AxB/1

== matlab function Boomerang_Simulink_Nav_Kalman/Newton's Equation/MATLAB Function1 ==
  data: udot input; u input; EULANGdot output; omega input; EULANG input
function EULANGdot = fcn(udot, u, omega, EULANG)
udotx = udot(1);
udoty = udot(2);

ux = u(1);
uy = u(2);

p = omega(1);
q = omega(2);
r = omega(3);

PHI = EULANG(1);
THETA = EULANG(2);

rn = r + (udoty*ux - udotx*uy)/(ux^2 + uy^2);
lambda = -tan(uy/ux);

PHIdot = (p*cos(lambda) - q*sin(lambda)) + (p*sin(lambda) + q*cos(lambda))*sin(PHI)*tan(THETA) + ...
    rn*cos(PHI)*tan(THETA);
THETAdot = (p*sin(lambda) + q*cos(lambda))*cos(PHI) - rn*sin(PHI);
PSIdot = (p*sin(lambda) + q*cos(lambda))*sin(PHI)/cos(THETA) + rn*cos(PHI)/cos(THETA);

EULANGdot = [PHIdot; THETAdot; PSIdot];

== matlab function Boomerang_Simulink_Nav_Kalman/Integration block1/MATLAB Function1 ==
  data: udot input; u input; EULANGdot output; omega input; EULANG input
function EULANGdot = fcn(udot, u, omega, EULANG)
udotx = udot(1);
udoty = udot(2);

ux = u(1);
uy = u(2);

p = omega(1);
q = omega(2);
r = omega(3);

PHI = EULANG(1);
THETA = EULANG(2);

rn = r + (udoty*ux - udotx*uy)/(ux^2 + uy^2);
lambda = -tan(uy/ux);

PHIdot = (p*cos(lambda) - q*sin(lambda)) + (p*sin(lambda) + q*cos(lambda))*sin(PHI)*tan(THETA) + ...
    rn*cos(PHI)*tan(THETA);
THETAdot = (p*sin(lambda) + q*cos(lambda))*cos(PHI) - rn*sin(PHI);
PSIdot = (p*sin(lambda) + q*cos(lambda))*sin(PHI)/cos(THETA) + rn*cos(PHI)/cos(THETA);

EULANGdot = [PHIdot; THETAdot; PSIdot];

== matlab function Boomerang_Simulink_Nav_Kalman/Navigation block/Body2Inertial ==
  data: r_nav input; R_nav output; EulAng input; invTI0 input
function R_nav  = fcn(r_nav, EulAng, invTI0)
phi = EulAng(1);
theta = EulAng(2);
psi = EulAng(3);

R01 = [
    1, 0, 0;
    0, cos(phi), sin(phi);
    0, -sin(phi), cos(phi)
    ];
R02 = [
    cos(theta), 0, -sin(theta);
    0, 1, 0;
    sin(theta), 0, cos(theta)
];
R03 = [
    cos(psi), sin(psi), 0;
    -sin(psi), cos(psi), 0;
    0, 0, 1
];
T0 = R01*R02*R03;
invT0 = transpose(T0);

R_nav = invTI0*invT0*r_nav;

== matlab function Boomerang_Simulink_Nav_Kalman/Navigation block/myStateTransitionFcn/Aerodynamics block/Aerodynamics ==
  settings: updateMethod=DISCRETE
  data: nw input; S input; Tj input; invTj input; x_ac input; l_integrate input; h input; rho input; c input; CLdata input; CDdata input; CMdata input; u input; omega input; v_wind input; TI0 input; EulAng input; FA output; thetaj input; MA output
function [FA, MA] = fcn(nw, S, Tj, invTj, x_ac, l_integrate, h, rho, c, CLdata, CDdata, CMdata,u, omega, v_wind, TI0, EulAng, thetaj)
% Initializing aerodynamic forces
FxjA = 0; 
FzjA = 0;
MxjA = 0;
MyjA = 0;
MzjA = 0;
rcrossF = [0;0;0];

phi = EulAng(1);
theta = EulAng(2);
psi = EulAng(3);

R01 = [
    1, 0, 0;
    0, cos(phi), sin(phi);
    0, -sin(phi), cos(phi)
    ];
R02 = [
    cos(theta), 0, -sin(theta);
    0, 1, 0;
    sin(theta), 0, cos(theta)
];
R03 = [
    cos(psi), sin(psi), 0;
    -sin(psi), cos(psi), 0;
    0, 0, 1
];
T0 = R01*R02*R03;

persistent flag FAz
if isempty(flag)
    flag = false;
    FAz = 0;
end

f = @(v_ind) v_ind - FAz/(2*rho*S*sqrt(u(1)^2 + (u(3)-v_ind)^2));
v_ind = fzero(f,0);

v_ind = [0; 0; -v_ind];

FA = [0; 0; 0];
MA = [0;0;0];

for i = 1:nw

    rA = @(eta) [x_ac; 0; 0] + invTj(:,:,i)*[0; eta; 0];
    
    w = @(eta) Tj(:,:,i)*( (-u-cross(omega, rA(eta))) - v_ind + T0*TI0*v_wind);
    
    % Function needed to select specific components from the w function handle
    g = @(a, x) a(x);
    alpha = @(eta) atan2(g(w(eta),3),g(w(eta),1)) + thetaj;
    w2 = @(eta) g(w(eta),1).^2 + g(w(eta),3).^2;
    
    % Piecewise linear fit for CL
    C_L = @(eta) interp1(CLdata(:,1), CLdata(:,2), alpha(eta), 'linear', 'extrap');
    
    % Piecewise linear fit for CD
    C_D = @(eta) interp1(CDdata(:,1), CDdata(:,2), alpha(eta), 'linear', 'extrap');
    
     % Piecewise linear fit for CM
    C_M = @(eta) interp1(CMdata(:,1), CMdata(:,2), alpha(eta), 'linear', 'extrap');

    l = @(eta) 0.5*rho*c*w2(eta)*C_L(eta);
    d = @(eta) 0.5*rho*c*w2(eta)*C_D(eta);
    m_eta = @(eta) 0.5*rho*w2(eta)*c^2*C_M(eta);

    int_funx = @(eta) -l(eta)*sin(alpha(eta)) + d(eta)*cos(alpha(eta));
    int_funz = @(eta) l(eta)*cos(alpha(eta)) + d(eta)*sin(alpha(eta));
    int_funMx = @(eta) (l(eta)*cos(alpha(eta)) + d(eta)*sin(alpha(eta)))*eta;
    int_funMy = @(eta) m_eta(eta); 
    int_funMz = @(eta) (l(eta)*sin(alpha(eta)) - d(eta)*cos(alpha(eta)))*eta;

    % Initializing the sum for using the trapezoidal integration method
    sumFxjA = 0; 
    sumFzjA = 0;
    sumMxjA = 0;
    sumMyjA = 0; 
    sumMzjA = 0; 
    
    % A for-loop is used for the sum as the MATLAB command ends up feeding
    % a vector as input to the int_fun, which ends up in errors
    for j = 2:(length(l_integrate)-1)
        sumFxjA = sumFxjA + int_funx(l_integrate(j));
        sumFzjA = sumFzjA + int_funz(l_integrate(j));
        sumMxjA = sumMxjA + int_funMx(l_integrate(j)); 
        sumMyjA = sumMyjA + int_funMy(l_integrate(j));
        sumMzjA = sumMzjA + int_funMz(l_integrate(j));
        FAetax = h/2*(int_funx(l_integrate(j-1)) + int_funx(l_integrate(j)));
        FAetaz = h/2*(int_funz(l_integrate(j-1)) + int_funz(l_integrate(j)));
        FAeta = invTj(:,:,i)*[FAetax; 0; FAetaz];
        rcrossF = rcrossF + cross(rA(l_integrate(j))+ invTj(:,:,i)*[0;h/2;0], FAeta);
    end

    % Explicitly written trapezoidal method - Trapz function does not work as functions like w require a scalar input
    FxjA = FxjA + h/2*(int_funx(l_integrate(1)) + 2*sumFxjA + ...
        int_funx(l_integrate(end)));  
    FzjA = FzjA + h/2*(int_funz(l_integrate(1)) + 2*sumFzjA + ...
        int_funz(l_integrate(end)));  
    FjA = [FxjA; 0; FzjA];
    FA = FA + invTj(:,:,i)*FjA;

    MxjA = MxjA + h/2*(int_funMx(l_integrate(1)) + 2*sumMxjA + ...
        int_funMx(l_integrate(end))); 
    MyjA = MyjA + h/2*(int_funMy(l_integrate(1)) + 2*sumMyjA + ...
        int_funMy(l_integrate(end))); 
    MzjA = MzjA + h/2*(int_funMz(l_integrate(1)) + 2*sumMzjA + ...
        int_funMz(l_integrate(end))); 
    MjA = [MxjA; MyjA; MzjA];

    MA = MA + invTj(:,:,i)*MjA + rcrossF;
end

FAz = FA(3);

== matlab function Boomerang_Simulink_Nav_Kalman/Navigation block/myStateTransitionFcn/EulerAngles/MATLAB Function ==
  data: omega input; EulRate output; phi input; theta input
function EulRate = fcn(omega, phi, theta)

phidot = omega(1) + omega(2)*sin(phi)*tan(theta) + omega(3)*cos(phi)*tan(theta);
thetadot = omega(2)*cos(phi) - omega(3)*sin(phi);
psidot = omega(2)*sin(phi)/cos(theta) + omega(3)*cos(phi)/cos(theta);

EulRate = [phidot; thetadot; psidot];

== matlab function Boomerang_Simulink_Nav_Kalman/Navigation block/myStateTransitionFcn/Gravity Force/MATLAB Function ==
  data: phi input; theta input; psi input; CG output; TI0 input
function CG = fcn(phi, theta, psi, TI0)
R01 = [
    1, 0, 0;
    0, cos(phi), sin(phi);
    0, -sin(phi), cos(phi)
    ];
R02 = [
    cos(theta), 0, -sin(theta);
    0, 1, 0;
    sin(theta), 0, cos(theta)
];
R03 = [
    cos(psi), sin(psi), 0;
    -sin(psi), cos(psi), 0;
    0, 0, 1
];
T0 = R01*R02*R03;

CG = T0*TI0*[0; 0; 1];

== matlab function Boomerang_Simulink_Nav_Kalman/Navigation block/myStateTransitionFcn/Newton's Equation/MATLAB Function1 ==
  data: udot input; u input; EULANGdot output; omega input; EULANG input
function EULANGdot = fcn(udot, u, omega, EULANG)
udotx = udot(1);
udoty = udot(2);

ux = u(1);
uy = u(2);

p = omega(1);
q = omega(2);
r = omega(3);

PHI = EULANG(1);
THETA = EULANG(2);

rn = r + (udoty*ux - udotx*uy)/(ux^2 + uy^2);
lambda = -tan(uy/ux);

PHIdot = (p*cos(lambda) - q*sin(lambda)) + (p*sin(lambda) + q*cos(lambda))*sin(PHI)*tan(THETA) + ...
    rn*cos(PHI)*tan(THETA);
THETAdot = (p*sin(lambda) + q*cos(lambda))*cos(PHI) - rn*sin(PHI);
PSIdot = (p*sin(lambda) + q*cos(lambda))*sin(PHI)/cos(THETA) + rn*cos(PHI)/cos(THETA);

EULANGdot = [PHIdot; THETAdot; PSIdot];

== matlab function Boomerang_Simulink_Nav_Kalman/Aerodynamics block/Aerodynamics ==
  settings: updateMethod=DISCRETE
  data: nw input; S input; Tj input; invTj input; x_ac input; l_integrate input; h input; rho input; c input; CLdata input; CDdata input; CMdata input; u input; omega input; v_wind input; TI0 input; EulAng input; FA output; thetaj input; MA output
function [FA, MA] = fcn(nw, S, Tj, invTj, x_ac, l_integrate, h, rho, c, CLdata, CDdata, CMdata,u, omega, v_wind, TI0, EulAng, thetaj)
% Initializing aerodynamic forces
FxjA = 0; 
FzjA = 0;
MxjA = 0;
MyjA = 0;
MzjA = 0;
rcrossF = [0;0;0];

phi = EulAng(1);
theta = EulAng(2);
psi = EulAng(3);

R01 = [
    1, 0, 0;
    0, cos(phi), sin(phi);
    0, -sin(phi), cos(phi)
    ];
R02 = [
    cos(theta), 0, -sin(theta);
    0, 1, 0;
    sin(theta), 0, cos(theta)
];
R03 = [
    cos(psi), sin(psi), 0;
    -sin(psi), cos(psi), 0;
    0, 0, 1
];
T0 = R01*R02*R03;

persistent flag FAz
if isempty(flag)
    flag = false;
    FAz = 0;
end

f = @(v_ind) v_ind - FAz/(2*rho*S*sqrt(u(1)^2 + (u(3)-v_ind)^2));
v_ind = fzero(f,0);

v_ind = [0; 0; -v_ind];

FA = [0; 0; 0];
MA = [0;0;0];

for i = 1:nw

    rA = @(eta) [x_ac; 0; 0] + invTj(:,:,i)*[0; eta; 0];
    
    w = @(eta) Tj(:,:,i)*( (-u-cross(omega, rA(eta))) - v_ind + T0*TI0*v_wind);
    
    % Function needed to select specific components from the w function handle
    g = @(a, x) a(x);
    alpha = @(eta) atan2(g(w(eta),3),g(w(eta),1)) + thetaj;
    w2 = @(eta) g(w(eta),1).^2 + g(w(eta),3).^2;
    
    % Piecewise linear fit for CL
    C_L = @(eta) interp1(CLdata(:,1), CLdata(:,2), alpha(eta), 'linear', 'extrap');
    
    % Piecewise linear fit for CD
    C_D = @(eta) interp1(CDdata(:,1), CDdata(:,2), alpha(eta), 'linear', 'extrap');
    
     % Piecewise linear fit for CM
    C_M = @(eta) interp1(CMdata(:,1), CMdata(:,2), alpha(eta), 'linear', 'extrap');

    l = @(eta) 0.5*rho*c*w2(eta)*C_L(eta);
    d = @(eta) 0.5*rho*c*w2(eta)*C_D(eta);
    m_eta = @(eta) 0.5*rho*w2(eta)*c^2*C_M(eta);

    int_funx = @(eta) -l(eta)*sin(alpha(eta)) + d(eta)*cos(alpha(eta));
    int_funz = @(eta) l(eta)*cos(alpha(eta)) + d(eta)*sin(alpha(eta));
    int_funMx = @(eta) (l(eta)*cos(alpha(eta)) + d(eta)*sin(alpha(eta)))*eta;
    int_funMy = @(eta) m_eta(eta); 
    int_funMz = @(eta) (l(eta)*sin(alpha(eta)) - d(eta)*cos(alpha(eta)))*eta;

    % Initializing the sum for using the trapezoidal integration method
    sumFxjA = 0; 
    sumFzjA = 0;
    sumMxjA = 0;
    sumMyjA = 0; 
    sumMzjA = 0; 
    
    % A for-loop is used for the sum as the MATLAB command ends up feeding
    % a vector as input to the int_fun, which ends up in errors
    for j = 2:(length(l_integrate)-1)
        sumFxjA = sumFxjA + int_funx(l_integrate(j));
        sumFzjA = sumFzjA + int_funz(l_integrate(j));
        sumMxjA = sumMxjA + int_funMx(l_integrate(j)); 
        sumMyjA = sumMyjA + int_funMy(l_integrate(j));
        sumMzjA = sumMzjA + int_funMz(l_integrate(j));
        FAetax = h/2*(int_funx(l_integrate(j-1)) + int_funx(l_integrate(j)));
        FAetaz = h/2*(int_funz(l_integrate(j-1)) + int_funz(l_integrate(j)));
        FAeta = invTj(:,:,i)*[FAetax; 0; FAetaz];
        rcrossF = rcrossF + cross(rA(l_integrate(j))+ invTj(:,:,i)*[0;h/2;0], FAeta);
    end

    % Explicitly written trapezoidal method - Trapz function does not work as functions like w require a scalar input
    FxjA = FxjA + h/2*(int_funx(l_integrate(1)) + 2*sumFxjA + ...
        int_funx(l_integrate(end)));  
    FzjA = FzjA + h/2*(int_funz(l_integrate(1)) + 2*sumFzjA + ...
        int_funz(l_integrate(end)));  
    FjA = [FxjA; 0; FzjA];
    FA = FA + invTj(:,:,i)*FjA;

    MxjA = MxjA + h/2*(int_funMx(l_integrate(1)) + 2*sumMxjA + ...
        int_funMx(l_integrate(end))); 
    MyjA = MyjA + h/2*(int_funMy(l_integrate(1)) + 2*sumMyjA + ...
        int_funMy(l_integrate(end))); 
    MzjA = MzjA + h/2*(int_funMz(l_integrate(1)) + 2*sumMzjA + ...
        int_funMz(l_integrate(end))); 
    MjA = [MxjA; MyjA; MzjA];

    MA = MA + invTj(:,:,i)*MjA + rcrossF;
end

FAz = FA(3);

== matlab function Boomerang_Simulink_Nav_Kalman/Gravity Force/MATLAB Function ==
  data: phi input; theta input; psi input; CG output; TI0 input
function CG = fcn(phi, theta, psi, TI0)
R01 = [
    1, 0, 0;
    0, cos(phi), sin(phi);
    0, -sin(phi), cos(phi)
    ];
R02 = [
    cos(theta), 0, -sin(theta);
    0, 1, 0;
    sin(theta), 0, cos(theta)
];
R03 = [
    cos(psi), sin(psi), 0;
    -sin(psi), cos(psi), 0;
    0, 0, 1
];
T0 = R01*R02*R03;

CG = T0*TI0*[0; 0; 1];

== matlab function Boomerang_Simulink_Nav_Kalman/Integration block/Body2Inertial ==
  data: u input; U output; EulAng input; invTI0 input
function U  = fcn(u, EulAng, invTI0)
phi = EulAng(1);
theta = EulAng(2);
psi = EulAng(3);

R01 = [
    1, 0, 0;
    0, cos(phi), sin(phi);
    0, -sin(phi), cos(phi)
    ];
R02 = [
    cos(theta), 0, -sin(theta);
    0, 1, 0;
    sin(theta), 0, cos(theta)
];
R03 = [
    cos(psi), sin(psi), 0;
    -sin(psi), cos(psi), 0;
    0, 0, 1
];
T0 = R01*R02*R03;
invT0 = transpose(T0);

U = invTI0*invT0*u;

== matlab function Boomerang_Simulink_Nav_Kalman/EulerAngles/MATLAB Function ==
  data: omega input; EulRate output; EulAng input
function EulRate = fcn(omega, EulAng)
phi = EulAng(1);
theta = EulAng(2);

phidot = omega(1) + omega(2)*sin(phi)*tan(theta) + omega(3)*cos(phi)*tan(theta);
thetadot = omega(2)*cos(phi) - omega(3)*sin(phi);
psidot = omega(2)*sin(phi)/cos(theta) + omega(3)*cos(phi)/cos(theta);

EulRate = [phidot; thetadot; psidot];

== matlab function Boomerang_Simulink_Nav_Kalman/Energy computation/Kinetic energy/Norm ==
  data: u input; y output
function y = fcn(u)

y = norm(u)^2;

== matlab function Boomerang_Simulink_Nav_Kalman/Integration block1/Body2Inertial ==
  data: u input; U output; phi input; theta input; psi input; invTI0 input
function U = fcn(u, phi, theta, psi, invTI0)
R01 = [
    1, 0, 0;
    0, cos(phi), sin(phi);
    0, -sin(phi), cos(phi)
    ];
R02 = [
    cos(theta), 0, -sin(theta);
    0, 1, 0;
    sin(theta), 0, cos(theta)
];
R03 = [
    cos(psi), sin(psi), 0;
    -sin(psi), cos(psi), 0;
    0, 0, 1
];
T0 = R01*R02*R03;
invT0 = transpose(T0);
U = invTI0*invT0*u;
